simulink model "statelessWriter2_2"  (Simulink 9.1)
settings: Solver=VariableStepAuto  StartTime=0.0  StopTime=100  RelTol=1e-3
settings Model: SuppressorTable=22 serialization::archive 11 0 6 0 0 0 0 0  Creator=root  LastModifiedBy=BEAR
settings DataIOCC: SaveFormat=Dataset
settings OptimizationCC: LifeSpan=auto
settings DebuggingCC: UnderspecifiedInitializationDetection=Simplified  MergeDetectMultiDrivingBlocksExec=error  SFUnexpectedBacktrackingDiag=error  SFNoUnconditionalDefaultTransitionDiag=error  SFExecutionAtInitializationDiag=warning
settings HardwareCC: ProdBitPerPointer=64  ProdBitPerSizeT=64  ProdBitPerPtrDiffT=64  ProdLargestAtomicFloat=Float  ProdIntDivRoundTo=Zero  ProdEndianess=LittleEndian  ProdWordSize=64  ProdHWDeviceType=Intel->x86-64 (Windows64)
settings ModelReferenceCC: PropagateSignalLabelsOutOfModel=on
settings GRTTargetCC: TargetLangStandard=C99 (ISO)  CombineOutputUpdateFcns=on  GRTInterface=off
settings ConfigComp: CovMetricSettings=dwe  CovHtmlReporting=off  CovSaveCumulativeToWorkspaceVar=off  CovSaveSingleToWorkspaceVar=off  CovExternalEMLEnable=on

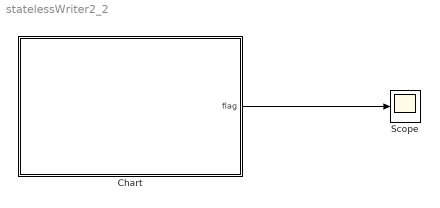
== system statelessWriter2_2 ==
  Chart : Stateflow chart  TreatAsAtomicUnit=on
  Scope : Scope
  wires:
  Chart/1(flag) -> Scope/1

== stateflow chart Chart ==
  settings: updateMethod=DISCRETE  sampleTime=2
  state repairing
    du: flag=0
  state waiting
    du: flag=1;
  state must_repair
    du: flag=1;
  repairing -> repairing [order 2] : [cansend==1]/{re_changes = re_changes - 1}
  must_repair -> repairing [order 1] : [after(5,sec)]
  must_repair -> must_repair [order 2] : [ACKNACK==1]/{re_changes = re_changes + 1}
  (default) -> waiting : {re_changes=0; ACKNACK=1; cansend=1}
  repairing -> waiting [order 1] : [re_changes==0]
  waiting -> must_repair [order 1] : [re_changes>0]{ACKNACK=0}
  waiting -> waiting [order 2] : [ACKNACK==1]/{re_changes = re_changes + 1}
  data: flag output double; re_changes local double; ResponseDelay constant double; cansend local double; ACKNACK local double
  events: event local FUNCTION_CALL_EVENT; event1 local FUNCTION_CALL_EVENT
